simulink model "MATLABFunction0"  (R2024b)
settings: Solver=ode4  StartTime=0.0  StopTime=600  FixedStep=0.01  RelTol=1e-3
settings Model: DVExtractedSubsystem=MATLAB Function  DVDesignModelName=simulation  Creator=simon  LastModifiedBy=simon
settings DebuggingCC: FrameProcessingCompatibilityMsg=none
settings RTWCC: TLCOptions=-aAlwaysIncludeCustomSrc=1

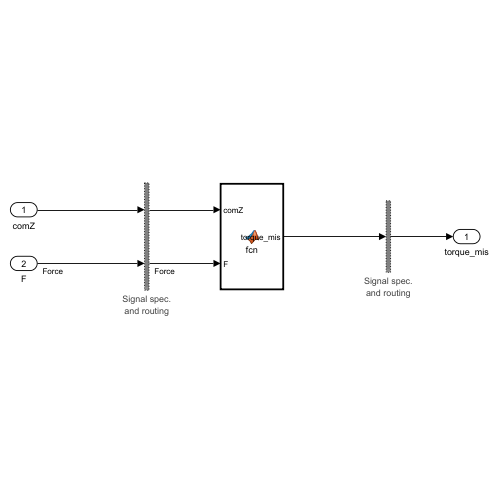
[thumbnail: Simulink's stored preview of the top-level diagram]
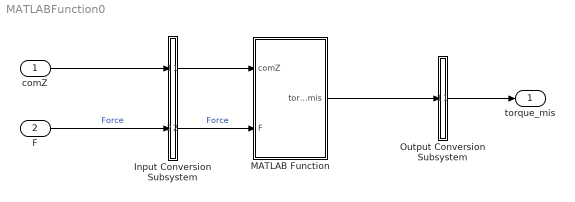
== system MATLABFunction0 ==
  comZ : Inport  OutDataTypeStr=double  PortDimensions=[1]  Interpolate=off
  F : Inport  Port=2  OutDataTypeStr=double  PortDimensions=[3, 1]  Interpolate=off
  Input Conversion Subsystem : Subsystem  Tag=__SLT_ICS__  Description=|
      | Signal spec.
      | and routing
      settings: AttributesFormatString=%<Description>
  MATLAB Function : MATLAB Function  TreatAsAtomicUnit=on
  Output Conversion Subsystem : Subsystem  Tag=__SLT_OCS__  Description=|
      | Signal spec.
      | and routing
      settings: AttributesFormatString=%<Description>
  torque_mis : Outport
  wires:
  comZ/1 -> Input Conversion Subsystem/1(Inport_1)
  F/1 -> Input Conversion Subsystem/2(Inport_2)  "Force"
  Output Conversion Subsystem/1(Outport_1) -> torque_mis/1
  Input Conversion Subsystem/1(Outport_1) -> MATLAB Function/1(comZ)
  Input Conversion Subsystem/2(Outport_2) -> MATLAB Function/2(F)  "Force"
  MATLAB Function/1(torque_mis) -> Output Conversion Subsystem/1(Inport_1)

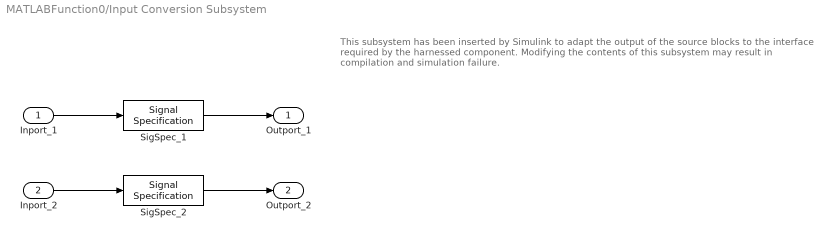
== system MATLABFunction0/Input Conversion Subsystem ==
  note: This subsystem has been inserted by Simulink to adapt the output of the source blocks to the interface required by the harnessed component.
      |  Modifying the contents of this subsystem may result in compilation and simulation failure.
  Inport_1 : Inport
  Inport_2 : Inport  Port=2
  SigSpec_1 : SignalSpecification  OutDataTypeStr=double  Dimensions=[1]
  SigSpec_2 : SignalSpecification  OutDataTypeStr=double  Dimensions=[3, 1]
  Outport_1 : Outport
  Outport_2 : Outport  Port=2
  wires:
  SigSpec_1/1 -> Outport_1/1
  Inport_1/1 -> SigSpec_1/1
  SigSpec_2/1 -> Outport_2/1
  Inport_2/1 -> SigSpec_2/1

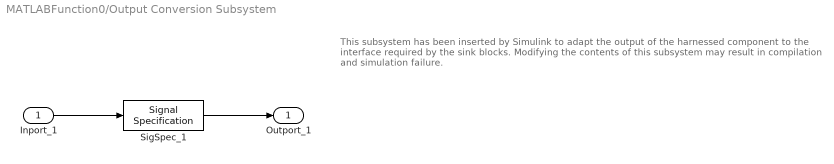
== system MATLABFunction0/Output Conversion Subsystem ==
  note: This subsystem has been inserted by Simulink to adapt the output of the harnessed component to the interface required by the sink blocks.
      |  Modifying the contents of this subsystem may result in compilation and simulation failure.
  Inport_1 : Inport
  SigSpec_1 : SignalSpecification  OutDataTypeStr=double  Dimensions=[3, 1]
  Outport_1 : Outport
  wires:
  Inport_1/1 -> SigSpec_1/1
  SigSpec_1/1 -> Outport_1/1

== matlab function MATLABFunction0/MATLAB Function ==
  data: comZ input; torque_mis output; F input
function torque_mis = fcn(comZ, F)

torque_mis = [F(1)*comZ; F(2)*comZ; 0];
